simulink model "LW_ctrl"  (R2024b)
settings: Solver=ode4  StartTime=0.0  StopTime=SIM_TIME  FixedStep=0.001  RelTol=1e-3  EnableMultiTasking=on
StartFcn:
  | %timestart = cputime;
StopFcn:
  | %dt = cputime - timestart
undefined symbols (not defined in the file or in its folder): AttCtrl_cycle, ControlMode, DEG2RAD, Earth, FlightMode, LW_ACRO_P_MAX, LW_ACRO_R_MAX, LW_ACRO_Y_MAX, LW_AERO_C0, LW_AERO_C1, LW_AERO_Y0, LW_ANGLE, LW_DMZ0, LW_DMZ_MIN, LW_LAT_CIRCLE, LW_MAN_PITCH_MAX, LW_MAN_ROLL_MAX, LW_MASS, LW_OB_CIRCLE_R, LW_OB_CIRCLE_V, LW_OB_CIRCLE_W, LW_OB_TYPE, LW_REX_YAW, LW_SERVOL_MAX, LW_SERVOR_MAX, LW_THR_HOVER, LW_WZ_MAX, LW_X_ACCEL_MAX, LW_X_ACCEL_MIN, LW_X_FF, LW_X_JERK_MAX, LW_X_P, LW_X_VEL_MAX, LW_Y_ACCEL_MAX, LW_Y_ACCEL_MIN, LW_Y_FF, LW_Y_JERK_MAX, LW_Y_P, LW_Y_VEL_MAX, LW_YAW_KAD, LW_YAW_KAP, LW_Z_ACCEL_LOW, LW_Z_ACCEL_UP, LW_Z_FF, LW_Z_JERK_MAX, LW_Z_P, LW_Z_VEL_MAX_UP, Map_xoffset, Map_yoffset, Map_zoffset, MAX_wdotx, MAX_wdoty, MAX_wdotz, Mixer_cycle, ModelParam_AccelMax, ModelParam_DelayAtt, ModelParam_DelayOmega, ModelParam_DelayPos, ModelParam_envAltitude, ModelParam_envGravityAcc ... (+57)
libraries: pixhawk_slib_uORB_RW x15, simulink x6, slpidlib x6, dspstat3 x5, aerolibnav x4, aerolibtransform2 x3, pixhawk_slib_sensors_actuators x2, etargetslib x2, pixhawk_slib_rfly x1, aerolibatmos2 x1, slrealtimeiplib x1, SignalEditorBlockLib x1
(part 2 of 6)

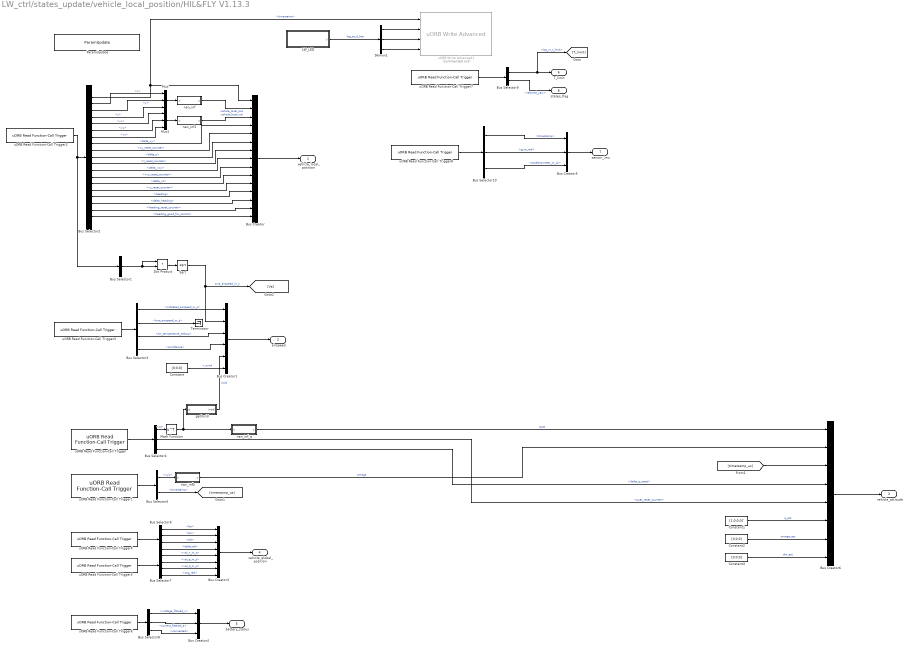
== system LW_ctrl/states_update/vehicle_local_position/HIL&FLY V1.13.3 ==
  Bus Creator : BusCreator  Inputs=15
  Bus Creator1 : BusCreator  Inputs=6
  Bus Creator3 : BusCreator  Inputs=8
  Bus Creator4 : BusCreator  Inputs=3
  Bus Creator5 : BusCreator  Inputs=3
  Bus Creator6 : BusCreator  Inputs=8
  Bus Selector1 : BusSelector  OutputSignals=vx,vy,vz  OutputAsBus=on
  Bus Selector10 : BusSelector  OutputSignals=timestamp,gyro_rad,accelerometer_m_s2
  Bus Selector2 : BusSelector  OutputSignals=timestamp,x,y,z,vx,vy,vz,delta_xy,xy_reset_counter,delta_z,z_reset_counter,delta_vxy,vxy_reset_counter,delta_vz,vz_reset_counter,heading,delta_heading,heading_reset_counter,heading_good_for_control
  Bus Selector3 : BusSelector  OutputSignals=indicated_airspeed_m_s,true_airspeed_m_s,air_temperature_celsius,confidence
  Bus Selector4 : BusSelector  OutputSignals=q,quat_reset_counter,delta_q_reset
  Bus Selector5 : BusSelector  OutputSignals=xyz,timestamp
  Bus Selector6 : BusSelector  OutputSignals=lat,lon,alt,delta_alt
  Bus Selector7 : BusSelector  OutputSignals=vel_n_m_s,vel_e_m_s,vel_d_m_s,cog_rad
  Bus Selector8 : BusSelector  OutputSignals=voltage_filtered_v,current_filtered_a,connected
  Bus Selector9 : BusSelector  OutputSignals=log_m_t_limit,relaxed_yaw
  Constant : Constant  Value=[0;0;0]  OutDataTypeStr=single
  Constant1 : Constant  Value=[1;0;0;0]'  OutDataTypeStr=single
  Constant2 : Constant  Value=[0;0;0]  OutDataTypeStr=single
  Constant3 : Constant  Value=[0;0;0]  OutDataTypeStr=single
  Demux1 : Demux  Outputs=3
  Dot Product : DotProduct  OutDataTypeStr=Inherit: Inherit via internal rule
  LW_LED : MATLAB Function  TreatAsAtomicUnit=on
  Math Function : Math  Operator=transpose
  Mux : Mux  Inputs=3
  Mux1 : Mux  Inputs=3
  ParamUpdate : pixhawk_slib_misc_utils/ParamUpdate  Description=|  Unformatted_StrSet=0  TLC_StrSet=0  NumParams=0  Ts=0
      | ParamUpdate Block
      | 
      | Use this block at your top-level of your model to insert a "parameter update" function in the generated code.
      settings: SourceProductName=Misc Utility Blocks
  Sqrt : Sqrt
  Terminator : Terminator
  getIncid : MATLAB Function  TreatAsAtomicUnit=on
  nan_inf : MATLAB Function  TreatAsAtomicUnit=on
  nan_inf0 : MATLAB Function  TreatAsAtomicUnit=on
  nan_inf1 : MATLAB Function  TreatAsAtomicUnit=on
  nan_inf_q : MATLAB Function  TreatAsAtomicUnit=on
  uORB Read Function-Call Trigger : pixhawk_slib_uORB_RW/uORB Read Function-Call Trigger  uORB_Topic_str='vehicle_attitude'  BusObjVar=Bus: vehicle_attitude_SL  uORB_Interval=0  AsyncOutput=off  Fcn_call_select=Generate Function Call Signal  TaskName='Task1'  Poll_timeout=100  Ts=-1
      settings: SourceProductName=uORB Read / Write Blocks
  uORB Read Function-Call Trigger1 : pixhawk_slib_uORB_RW/uORB Read Function-Call Trigger  uORB_Topic_str='vehicle_angular_velocity'  BusObjVar=Bus: vehicle_angular_velocity_SL  uORB_Interval=0  AsyncOutput=off  Fcn_call_select=Generate Function Call Signal  TaskName='Task1'  Poll_timeout=100  Ts=-1
      settings: SourceProductName=uORB Read / Write Blocks
  uORB Read Function-Call Trigger2 : pixhawk_slib_uORB_RW/uORB Read Function-Call Trigger  Priority=2  uORB_Topic_str='vehicle_local_position'  BusObjVar=Bus: vehicle_local_position_SL  uORB_Interval=0  AsyncOutput=off  Fcn_call_select=Generate Function Call Signal  TaskName='Task2'  Poll_timeout=20  Ts=-1
      settings: SourceProductName=uORB Read / Write Blocks
  uORB Read Function-Call Trigger3 : pixhawk_slib_uORB_RW/uORB Read Function-Call Trigger  Priority=2  uORB_Topic_str='airspeed'  BusObjVar=Bus: airspeed_SL  uORB_Interval=0  AsyncOutput=off  Fcn_call_select=Generate Function Call Signal  TaskName='Task2'  Poll_timeout=20  Ts=-1
      settings: SourceProductName=uORB Read / Write Blocks
  uORB Read Function-Call Trigger4 : pixhawk_slib_uORB_RW/uORB Read Function-Call Trigger  Priority=2  uORB_Topic_str='vehicle_global_position'  BusObjVar=Bus: vehicle_global_position_SL  uORB_Interval=0  AsyncOutput=off  Fcn_call_select=Generate Function Call Signal  TaskName='Task2'  Poll_timeout=20  Ts=-1
      settings: SourceProductName=uORB Read / Write Blocks
  uORB Read Function-Call Trigger5 : pixhawk_slib_uORB_RW/uORB Read Function-Call Trigger  Priority=2  uORB_Topic_str='vehicle_gps_position'  BusObjVar=Bus: vehicle_gps_position_SL  uORB_Interval=0  AsyncOutput=off  Fcn_call_select=Generate Function Call Signal  TaskName='Task2'  Poll_timeout=20  Ts=-1
      settings: SourceProductName=uORB Read / Write Blocks
  uORB Read Function-Call Trigger6 : pixhawk_slib_uORB_RW/uORB Read Function-Call Trigger  Priority=2  uORB_Topic_str='battery_status'  BusObjVar=Bus: battery_status_SL  uORB_Interval=0  AsyncOutput=off  Fcn_call_select=Generate Function Call Signal  TaskName='Task2'  Poll_timeout=20  Ts=-1
      settings: SourceProductName=uORB Read / Write Blocks
  uORB Read Function-Call Trigger7 : pixhawk_slib_uORB_RW/uORB Read Function-Call Trigger  Priority=2  uORB_Topic_str='costom_lw_mixer'  BusObjVar=Bus: costom_lw_mixer_SL  uORB_Interval=0  AsyncOutput=off  Fcn_call_select=Generate Function Call Signal  TaskName='Task2'  Poll_timeout=20  Ts=-1
      settings: SourceProductName=uORB Read / Write Blocks
  uORB Read Function-Call Trigger8 : pixhawk_slib_uORB_RW/uORB Read Function-Call Trigger  Priority=2  uORB_Topic_str='sensor_combined'  BusObjVar=Bus: sensor_combined_SL  uORB_Interval=0  AsyncOutput=off  Fcn_call_select=Generate Function Call Signal  TaskName='Task2'  Poll_timeout=20  Ts=-1
      settings: SourceProductName=uORB Read / Write Blocks
  uORB Write Advanced1 : pixhawk_slib_uORB_RW/uORB Write Advanced  Commented=on  Ts=0  uORB_AdvtQueue=on  uORB_FieldEnabledArr="0  0  0  1  0  0  0  0  0  0  0"  uORB_Topic_str=0  uORB_Struct_DT="[1  1  1  1  1]"  BlockInputCount=5  uORB_StructParams="[\"voltage_v\",\"voltage_filtered_v\",\"current_a\",\"current_filtered_a\",\"remaining\"]"  uORB_PortSizes="[1  1  1  1]"  MsgSizeOf=0  MW_update=true
      settings: SourceProductName=uORB Read / Write Blocks
  vehicle_local_position : Outport  VectorParamsAs1DForOutWhenUnconnected=off
  airspeed : Outport  Port=2  VectorParamsAs1DForOutWhenUnconnected=off
  vehicle_attitude : Outport  Port=3  VectorParamsAs1DForOutWhenUnconnected=off
  vehicle_global_position : Outport  Port=4  OutDataTypeStr=Bus: vehicle_global_position_bus  VectorParamsAs1DForOutWhenUnconnected=off
  battery_status : Outport  Port=5  OutDataTypeStr=Bus: battery_status_bus  VectorParamsAs1DForOutWhenUnconnected=off
  T_limit : Outport  Port=6  VectorParamsAs1DForOutWhenUnconnected=off
  sensor_imu : Outport  Port=7  VectorParamsAs1DForOutWhenUnconnected=off
  states_flag : Outport  Port=8  VectorParamsAs1DForOutWhenUnconnected=off
  wires:
  Bus Selector1/1 -> Dot Product/1, Dot Product/2
  Bus Selector2/6 -> Mux1/2  "<vy>"
  Bus Selector2/3 -> Mux/2  "<y>"
  uORB Read Function-Call Trigger2/1 -> Bus Selector1/1, Bus Selector2/1
  uORB Read Function-Call Trigger3/1 -> Bus Selector3/1
  Sqrt/1 -> Bus Creator1/2, [Va]  "true_airspeed_m_s"
  Bus Selector2/2 -> Mux/1  "<x>"
  Bus Selector8/1 -> Bus Creator4/1  "<voltage_filtered_v>"
  Bus Selector10/1 -> Bus Creator5/1  "<timestamp>"
  Bus Selector7/1 -> Bus Creator3/5  "<vel_n_m_s>"
  Dot Product/1 -> Sqrt/1
  Mux/1 -> nan_inf/1(u)
  Bus Creator5/1 -> sensor_imu/1
  Bus Selector10/3 -> Bus Creator5/3  "<accelerometer_m_s2>"
  uORB Read Function-Call Trigger6/1 -> Bus Selector8/1
  Bus Selector2/4 -> Mux/3  "<z>"
  Bus Creator/1 -> vehicle_local_position/1
  Bus Selector6/3 -> Bus Creator3/3  "<alt>"
  Bus Selector10/2 -> Bus Creator5/2  "<gyro_rad>"
  Bus Selector9/1 -> [T_limit], T_limit/1  "<log_m_t_limit>"
  Constant/1 -> Bus Creator1/6  "v_wind"
  Mux1/1 -> nan_inf1/1(u)
  nan_inf/1(y) -> Bus Creator/2  "vehicle_local_pos"
  Bus Selector7/3 -> Bus Creator3/7  "<vel_d_m_s>"
  uORB Read Function-Call Trigger5/1 -> Bus Selector7/1
  Bus Selector2/5 -> Mux1/1  "<vx>"
  uORB Read Function-Call Trigger4/1 -> Bus Selector6/1
  uORB Read Function-Call Trigger8/1 -> Bus Selector10/1
  Bus Selector6/1 -> Bus Creator3/1  "<lat>"
  Bus Selector2/7 -> Mux1/3  "<vz>"
  Bus Selector8/3 -> Bus Creator4/3  "<connected>"
  getIncid/1(incid) -> Bus Creator1/5  "incid"
  Bus Selector4/1 -> Math Function/1  "<q>"
  Bus Selector6/4 -> Bus Creator3/4  "<delta_alt>"
  nan_inf_q/1(y) -> Bus Creator6/1  "quat"
  Bus Selector7/4 -> Bus Creator3/8  "<cog_rad>"
  uORB Read Function-Call Trigger1/1 -> Bus Selector5/1
  Bus Creator1/1 -> airspeed/1
  Bus Selector3/3 -> Bus Creator1/3  "<air_temperature_celsius>"
  Bus Selector5/1 -> nan_inf0/1(u)  "<xyz>"
  Math Function/1 -> getIncid/1(q), nan_inf_q/1(u)
  Bus Selector6/2 -> Bus Creator3/2  "<lon>"
  Bus Creator3/1 -> vehicle_global_position/1
  Bus Selector7/2 -> Bus Creator3/6  "<vel_e_m_s>"
  Bus Selector9/2 -> states_flag/1  "<relaxed_yaw>"
  Bus Selector3/1 -> Bus Creator1/1  "<indicated_airspeed_m_s>"
  Bus Creator4/1 -> battery_status/1
  Bus Selector8/2 -> Bus Creator4/2  "<current_filtered_a>"
  uORB Read Function-Call Trigger/1 -> Bus Selector4/1
  nan_inf1/1(y) -> Bus Creator/3  "vehicle_local_vel"
  uORB Read Function-Call Trigger7/1 -> Bus Selector9/1
  Bus Selector5/2 -> [timestamp_us]  "<timestamp>"
  Bus Selector3/2 -> Terminator/1  "<true_airspeed_m_s>"
  Bus Selector3/4 -> Bus Creator1/4  "<confidence>"
  Bus Selector2/1 -> Bus Creator/1, uORB Write Advanced1/1  "<timestamp>"
  Demux1/2 -> uORB Write Advanced1/3
  Demux1/3 -> uORB Write Advanced1/4
  Demux1/1 -> uORB Write Advanced1/2
  LW_LED/1(y) -> Demux1/1  "log_ac_d_hat"
  Bus Selector2/8 -> Bus Creator/4  "<delta_xy>"
  Bus Selector2/9 -> Bus Creator/5  "<xy_reset_counter>"
  Bus Selector2/10 -> Bus Creator/6  "<delta_z>"
  Bus Selector2/11 -> Bus Creator/7  "<z_reset_counter>"
  Bus Selector2/12 -> Bus Creator/8  "<delta_vxy>"
  Bus Selector2/13 -> Bus Creator/9  "<vxy_reset_counter>"
  Bus Selector2/14 -> Bus Creator/10  "<delta_vz>"
  Bus Selector2/15 -> Bus Creator/11  "<vz_reset_counter>"
  Bus Selector2/16 -> Bus Creator/12  "<heading>"
  Bus Selector2/17 -> Bus Creator/13  "<delta_heading>"
  Bus Selector2/18 -> Bus Creator/14  "<heading_reset_counter>"
  Bus Selector2/19 -> Bus Creator/15  "<heading_good_for_control>"
  [timestamp_us] -> Bus Creator6/3
  Bus Creator6/1 -> vehicle_attitude/1
  Bus Selector4/2 -> Bus Creator6/5  "<quat_reset_counter>"
  nan_inf0/1(y) -> Bus Creator6/2  "omega"
  Bus Selector4/3 -> Bus Creator6/4  "<delta_q_reset>"
  Constant1/1 -> Bus Creator6/6  "q_est"
  Constant2/1 -> Bus Creator6/7  "omega_est"
  Constant3/1 -> Bus Creator6/8  "dm_est"

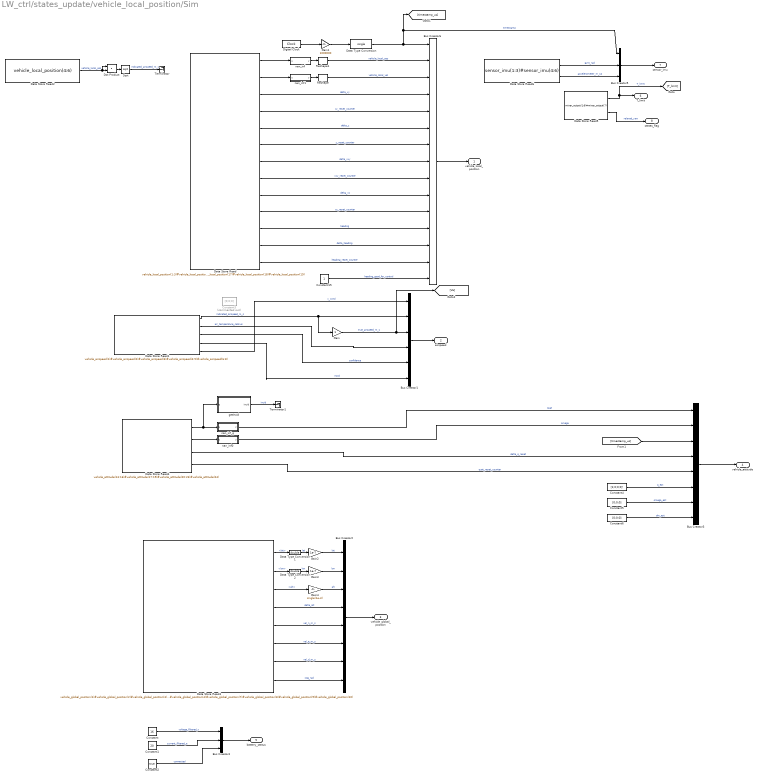
== system LW_ctrl/states_update/vehicle_local_position/Sim ==
  Bus Creator1 : BusCreator  Inputs=6
  Bus Creator2 : BusCreator  Inputs=8
  Bus Creator3 : BusCreator  Inputs=8
  Bus Creator4 : BusCreator  Inputs=3
  Bus Creator5 : BusCreator  Inputs=3
  Bus Creator6 : BusCreator  Inputs=15
  Constant : Constant  Value=16  OutDataTypeStr=single
  Constant1 : Constant  Value=20  OutDataTypeStr=single
  Constant15 : Constant  OutDataTypeStr=boolean
  Constant2 : Constant  Value=true  OutDataTypeStr=boolean
  Constant3 : Constant  Commented=on  Value=[0;0;0]  OutDataTypeStr=single
  Constant4 : Constant  Value=[1;0;0;0]'  OutDataTypeStr=single
  Constant5 : Constant  Value=[0;0;0]  OutDataTypeStr=single
  Constant6 : Constant  Value=[0;0;0]  OutDataTypeStr=single
  Data Store Read : DataStoreRead  DataStoreName=vehicle_local_position  DataStoreElements=vehicle_local_position(1:3)#vehicle_local_position(4:6)#vehicle_local_position(7:8)#vehicle_local_position(9)#vehicle_local_position(10)#vehicle_local_position(11)#vehicle_local_position(12:13)#vehicle_local_position(14)#vehicle_local_position(15)#vehicle_local_position(16)#vehicle_local_position(17)#vehicle_local_position(18)#vehicle_local_position(19)  IndexOptions=Index vector (dialog)  Indices=1  OutputSizes=1
  Data Store Read1 : DataStoreRead  DataStoreName=vehicle_airspeed  DataStoreElements=vehicle_airspeed(1)#vehicle_airspeed(2)#vehicle_airspeed(3)#vehicle_airspeed(4:5)#vehicle_airspeed(6:8)  IndexOptions=Index vector (dialog)  Indices=1  OutputSizes=1
  Data Store Read2 : DataStoreRead  DataStoreName=vehicle_local_position  DataStoreElements=vehicle_local_position(4:6)  IndexOptions=Index vector (dialog)  Indices=1  OutputSizes=1
  Data Store Read3 : DataStoreRead  DataStoreName=vehicle_global_position  DataStoreElements=vehicle_global_position(1)#vehicle_global_position(2)#vehicle_global_position(3)#vehicle_global_position(4)#vehicle_global_position(7)#vehicle_global_position(8)#vehicle_global_position(9)#vehicle_global_position(10)  IndexOptions=Index vector (dialog)  Indices=1  OutputSizes=1
  Data Store Read4 : DataStoreRead  DataStoreName=vehicle_attitude  DataStoreElements=vehicle_attitude(13:16)#vehicle_attitude(17:19)#vehicle_attitude(20:23)#vehicle_attitude(24)  IndexOptions=Index vector (dialog)  Indices=1  OutputSizes=1
  Data Store Read5 : DataStoreRead  Description=|  DataStoreName=mixer_output  DataStoreElements=mixer_output(1:6)#mixer_output(7)  IndexOptions=Index vector (dialog)  Indices=1  OutputSizes=1
      | 1-4:motor command
      | 5-6:aileron command
  Data Store Read6 : DataStoreRead  DataStoreName=sensor_imu  DataStoreElements=sensor_imu(1:3)#sensor_imu(4:6)  IndexOptions=Index vector (dialog)  Indices=1  OutputSizes=1
  Data Type Conversion : DataTypeConversion  OutDataTypeStr=single  SaturateOnIntegerOverflow=off  RndMeth=Floor
  Data Type Conversion1 : DataTypeConversion  OutDataTypeStr=double  SaturateOnIntegerOverflow=off  RndMeth=Floor
  Data Type Conversion2 : DataTypeConversion  OutDataTypeStr=double  SaturateOnIntegerOverflow=off  RndMeth=Floor
  Digital Clock : DigitalClock  SampleTime=-1
  Dot Product : DotProduct  OutDataTypeStr=Inherit: Inherit via internal rule
  Gain : Gain
  Gain1 : Gain  Gain=1000000
  Gain2 : Gain  Gain=1e-7  OutDataTypeStr=double
  Gain3 : Gain  Gain=1e-7  OutDataTypeStr=double
  Gain4 : Gain  Gain=single(1e-3)  OutDataTypeStr=single
  Reshape : Reshape  OutputDimensionality=Column vector (2-D)
  Reshape1 : Reshape  OutputDimensionality=Column vector (2-D)
  Sqrt : Sqrt
  Terminator : Terminator
  Terminator1 : Terminator
  getIncid : MATLAB Function  TreatAsAtomicUnit=on
  nan_inf : MATLAB Function  TreatAsAtomicUnit=on
  nan_inf0 : MATLAB Function  TreatAsAtomicUnit=on
  nan_inf1 : MATLAB Function  TreatAsAtomicUnit=on
  nan_inf_q : MATLAB Function  TreatAsAtomicUnit=on
  vehicle_local_position : Outport  VectorParamsAs1DForOutWhenUnconnected=off
  airspeed : Outport  Port=2  VectorParamsAs1DForOutWhenUnconnected=off
  vehicle_global_position : Outport  Port=3  OutDataTypeStr=Bus: vehicle_global_position_bus  VectorParamsAs1DForOutWhenUnconnected=off
  vehicle_attitude : Outport  Port=4  VectorParamsAs1DForOutWhenUnconnected=off
  battery_status : Outport  Port=5  OutDataTypeStr=Bus: battery_status_bus  VectorParamsAs1DForOutWhenUnconnected=off
  T_limit : Outport  Port=6  VectorParamsAs1DForOutWhenUnconnected=off
  sensor_imu : Outport  Port=7  VectorParamsAs1DForOutWhenUnconnected=off
  states_flag : Outport  Port=8  VectorParamsAs1DForOutWhenUnconnected=off
  wires:
  Data Store Read/1 -> nan_inf/1(u)
  Data Store Read/2 -> nan_inf1/1(u)
  nan_inf/1(y) -> Reshape1/1
  nan_inf1/1(y) -> Reshape/1
  Digital Clock/1 -> Gain1/1
  Reshape/1 -> Bus Creator6/3  "vehicle_local_vel"
  Reshape1/1 -> Bus Creator6/2  "vehicle_local_pos"
  Data Store Read1/3 -> Bus Creator1/5  "confidence"
  Data Store Read1/2 -> Bus Creator1/4  "air_temperature_celsius"
  Data Store Read2/1 -> Dot Product/2, Dot Product/1  "vehicle_local_pos"
  Dot Product/1 -> Sqrt/1
  Sqrt/1 -> Terminator/1  "indicated_airspeed_m_s"
  Gain/1 -> [Va], Bus Creator1/3  "true_airspeed_m_s"
  Bus Creator1/1 -> airspeed/1
  Data Store Read1/1 -> Bus Creator1/2, Gain/1  "indicated_airspeed_m_s"
  Data Store Read3/5 -> Bus Creator2/5  "vel_n_m_s"
  Gain3/1 -> Bus Creator2/2  "lon"
  Gain2/1 -> Bus Creator2/1  "lat"
  Data Store Read3/8 -> Bus Creator2/8  "cog_rad"
  Data Store Read3/3 -> Gain4/1  "<alt>"
  Data Store Read3/4 -> Bus Creator2/4  "delta_alt"
  Data Store Read3/6 -> Bus Creator2/6  "vel_e_m_s"
  Data Store Read3/1 -> Data Type Conversion1/1  "<lat>"
  Data Store Read3/7 -> Bus Creator2/7  "vel_d_m_s"
  Bus Creator2/1 -> vehicle_global_position/1
  Gain4/1 -> Bus Creator2/3  "alt"
  Data Store Read3/2 -> Data Type Conversion2/1  "<lon>"
  Data Store Read4/1 -> nan_inf_q/1(u), getIncid/1(q)
  Bus Creator3/1 -> vehicle_attitude/1
  Data Store Read4/2 -> nan_inf0/1(u)
  Data Store Read1/4 -> Bus Creator1/6  "incid"
  Gain1/1 -> Data Type Conversion/1
  Data Type Conversion1/1 -> Gain2/1  "lat"
  Data Type Conversion2/1 -> Gain3/1  "lon"
  getIncid/1(incid) -> Terminator1/1  "incid"
  Constant1/1 -> Bus Creator4/2  "current_filtered_a"
  Constant/1 -> Bus Creator4/1  "voltage_filtered_v"
  Bus Creator4/1 -> battery_status/1
  Constant2/1 -> Bus Creator4/3  "connected"
  Data Store Read5/1 -> [T_limit], T_limit/1  "T_limit"
  Data Store Read1/5 -> Bus Creator1/1  "v_wind"
  Bus Creator5/1 -> sensor_imu/1
  Data Store Read6/2 -> Bus Creator5/3  "accelerometer_m_s2"
  Data Store Read6/1 -> Bus Creator5/2  "gyro_rad"
  Data Type Conversion/1 -> [timestamp_us], Bus Creator5/1, Bus Creator6/1  "timestamp"
  Data Store Read5/2 -> states_flag/1  "relaxed_yaw"
  Data Store Read/4 -> Bus Creator6/5  "xy_reset_counter"
  Data Store Read/3 -> Bus Creator6/4  "delta_xy"
  Data Store Read/9 -> Bus Creator6/10  "delta_vz"
  Data Store Read/5 -> Bus Creator6/6  "delta_z"
  Data Store Read/12 -> Bus Creator6/13  "delta_heading"
  Data Store Read/13 -> Bus Creator6/14  "heading_reset_counter"
  Data Store Read/11 -> Bus Creator6/12  "heading"
  Data Store Read/6 -> Bus Creator6/7  "z_reset_counter"
  Constant15/1 -> Bus Creator6/15  "heading_good_for_control"
  Data Store Read/10 -> Bus Creator6/11  "vz_reset_counter"
  Data Store Read/8 -> Bus Creator6/9  "vxy_reset_counter"
  Data Store Read/7 -> Bus Creator6/8  "delta_vxy"
  Bus Creator6/1 -> vehicle_local_position/1
  Data Store Read4/3 -> Bus Creator3/4  "delta_q_reset"
  nan_inf0/1(y) -> Bus Creator3/2  "omega"
  Data Store Read4/4 -> Bus Creator3/5  "quat_reset_counter"
  nan_inf_q/1(y) -> Bus Creator3/1  "quat"
  [timestamp_us] -> Bus Creator3/3
  Constant6/1 -> Bus Creator3/8  "dm_est"
  Constant4/1 -> Bus Creator3/6  "q_est"
  Constant5/1 -> Bus Creator3/7  "omega_est"

== system LW_ctrl/Controller/PID_Controller/PID_Controller/altitude control ==
  p : Inport
  q : Inport  Port=2
  attitude_d : Inport  Port=3
  r : Inport  Port=4
  f_d : Inport  Port=5
  quat : Inport  Port=6
  vehicle_mode : Inport  Port=7
  Bus Selector3 : BusSelector  OutputSignals=flight_mode,arm,ctrl_mode
  Cast To Single : DataTypeConversion  OutDataTypeStr=single  SaturateOnIntegerOverflow=off  RndMeth=Floor
  MATLAB Function : MATLAB Function
  MATLAB Function1 : MATLAB Function
  Mux12 : Mux
  Output_Limits1 : Saturate  UpperLimit=15  LowerLimit=0
  Selector1 : Selector  InputPortWidth=3  IndexOptions=Index vector (dialog)  Indices=[1]  OutputSizes=1
  Selector2 : Selector  InputPortWidth=3  IndexOptions=Index vector (dialog)  Indices=3  OutputSizes=1
  Selector3 : Selector  InputPortWidth=3  IndexOptions=Index vector (dialog)  Indices=2  OutputSizes=1
  Sum : Sum  Inputs=|+-
  Sum2 : Sum  Inputs=|+-
  Sum3 : Sum  Inputs=|+-
  attrates_ref_selector : MATLAB Function  TreatAsAtomicUnit=on
  wx_control : slpidlib/PID Controller  Controller=PID  Form=Parallel  TimeDomain=Discrete-time  UseExternalTs=off  SampleTime=-1  IntegratorMethod=Forward Euler  FilterMethod=Forward Euler  ControllerParametersSource=internal  P=20  I=0  UseKiTs=off  D=0  UseExternalDerivativeSource=off  N=100  UseFilter=on  TunerSelectOption=Transfer Function Based (PID Tuner App)  InitialConditionSource=internal  InitialConditionForIntegrator=0  InitialConditionForFilter=0  DifferentiatorICPrevScaledInput=0  ExternalReset=level  TrackingMode=off  Kt=1  LimitOutput=on  SatLimitsSource=internal  UpperSaturationLimit=MAX_wdotx  LowerSaturationLimit=-MAX_wdotx  LinearizeAsGain=off  AntiWindupMode=clamping  Kb=1  LimitIntegrator=off  UpperIntegratorSaturationLimit=inf  LowerIntegratorSaturationLimit=-inf  POutMin=[]  POutMax=[]  IOutMin=[]  IOutMax=[]  DOutMin=[]  DOutMax=[]  NOutMin=[]  NOutMax=[]  SumOutMin=[]  SumOutMax=[]  SaturationOutMin=[]  SaturationOutMax=[]  PParamMin=[]  PParamMax=[]  IParamMin=[]  IParamMax=[]  DParamMin=[]  DParamMax=[]  NParamMin=[]  NParamMax=[]  KbParamMin=[]  KbParamMax=[]  KtParamMin=[]  KtParamMax=[]  KbOutMin=[]  KbOutMax=[]  KtOutMin=[]  KtOutMax=[]  IntegratorOutMin=Saturation_I_Wx_Low  IntegratorOutMax=Saturation_I_Wx_Up  FilterOutMin=[]  FilterOutMax=[]  SumI1OutMin=[]  SumI1OutMax=[]  SumI2OutMin=[]  SumI2OutMax=[]  SumI3OutMin=[]  SumI3OutMax=[]  SumI4OutMin=[]  SumI4OutMax=[]  SumDOutMin=[]  SumDOutMax=[]  DifferentiatorOutMin=[]  DifferentiatorOutMax=[]  FilterDiffOutCoefMin=[]  FilterDiffOutCoefMax=[]  ReciprocalOutMin=[]  ReciprocalOutMax=[]  SumDenOutMin=[]  SumDenOutMax=[]  SumNumOutMin=[]  SumNumOutMax=[]  DivideOutMin=[]  DivideOutMax=[]  UdiffTsProdOutMin=[]  UdiffTsProdOutMax=[]  NTsProdOutMin=[]  NTsProdOutMax=[]  UintegralTsProdOutMin=[]  UintegralTsProdOutMax=[]  UngainTsProdOutMin=[]  UngainTsProdOutMax=[]  ClampingZeroOutDataTypeStr=Inherit: Inherit via back propagation  ClampingZeroOutMin=[]  ClampingZeroOutMax=[]  FilterDenConstantOutDataTypeStr=Inherit: Inherit via back propagation  FilterDenConstantOutMin=[]  FilterDenConstantOutMax=[]  PCopyOutDataTypeStr=Inherit: Inherit via back propagation  PCopyOutMin=[]  PCopyOutMax=[]  NCopyOutDataTypeStr=Inherit: Inherit via back propagation  NCopyOutMin=[]  NCopyOutMax=[]  IntegratorContinuousStateAttributes=''  IntegratorStateMustResolveToSignalObject=off  IntegratorRTWStateStorageClass=Auto  FilterContinuousStateAttributes=''  FilterStateMustResolveToSignalObject=off  FilterRTWStateStorageClass=Auto  ParallelPVariant=InternalParameters  IdealPVariant=Disabled  IVariant=InternalParameters  DVariant=InternalParameters  IntegratorVariant=Discrete  SatVariant=Enabled  AWVariant=DiscClampingParallel  PCopyVariant=Disabled  TRVariant=Disabled  FdbkBlocksVariant=Forward  IdealPFdbkVariant=Disabled  SatFdbkVariant=Disabled  DerivativeFilterVariant=ForwardEulerFilter  NVariant=InternalParameters  NCopyVariant=Disabled  FilterICVariant=InternalICsFilter  IntegratorICVariant=InternalICs  ExternalResetVariant=ExternalReset  TRSumVariant=Passthrough  SumFdbkVariant=Disabled  SumVariant=Sum_PID  TsampFilterVariant=InternalTs  TsampNgainVariant=Passthrough  TsampIntegralVariant=Disabled_SignalSpec  ExternalSaturationOutDataTypeStr=Inherit: Same as second input  DerivativeSourceVariant=ErrorSignal  PreIntVariant=InternalPreInt
  wy_control : slpidlib/PID Controller  Controller=PID  Form=Parallel  TimeDomain=Discrete-time  UseExternalTs=off  SampleTime=-1  IntegratorMethod=Forward Euler  FilterMethod=Forward Euler  ControllerParametersSource=internal  P=20  I=0  UseKiTs=off  D=0  UseExternalDerivativeSource=off  N=100  UseFilter=on  TunerSelectOption=Transfer Function Based (PID Tuner App)  InitialConditionSource=internal  InitialConditionForIntegrator=0  InitialConditionForFilter=0  DifferentiatorICPrevScaledInput=0  ExternalReset=level  TrackingMode=off  Kt=1  LimitOutput=on  SatLimitsSource=internal  UpperSaturationLimit=MAX_wdoty  LowerSaturationLimit=-MAX_wdoty  LinearizeAsGain=off  AntiWindupMode=clamping  Kb=1  LimitIntegrator=off  UpperIntegratorSaturationLimit=inf  LowerIntegratorSaturationLimit=-inf  POutMin=[]  POutMax=[]  IOutMin=[]  IOutMax=[]  DOutMin=[]  DOutMax=[]  NOutMin=[]  NOutMax=[]  SumOutMin=[]  SumOutMax=[]  SaturationOutMin=[]  SaturationOutMax=[]  PParamMin=[]  PParamMax=[]  IParamMin=[]  IParamMax=[]  DParamMin=[]  DParamMax=[]  NParamMin=[]  NParamMax=[]  KbParamMin=[]  KbParamMax=[]  KtParamMin=[]  KtParamMax=[]  KbOutMin=[]  KbOutMax=[]  KtOutMin=[]  KtOutMax=[]  IntegratorOutMin=Saturation_I_Wy_Low  IntegratorOutMax=Saturation_I_Wy_Up  FilterOutMin=[]  FilterOutMax=[]  SumI1OutMin=[]  SumI1OutMax=[]  SumI2OutMin=[]  SumI2OutMax=[]  SumI3OutMin=[]  SumI3OutMax=[]  SumI4OutMin=[]  SumI4OutMax=[]  SumDOutMin=[]  SumDOutMax=[]  DifferentiatorOutMin=[]  DifferentiatorOutMax=[]  FilterDiffOutCoefMin=[]  FilterDiffOutCoefMax=[]  ReciprocalOutMin=[]  ReciprocalOutMax=[]  SumDenOutMin=[]  SumDenOutMax=[]  SumNumOutMin=[]  SumNumOutMax=[]  DivideOutMin=[]  DivideOutMax=[]  UdiffTsProdOutMin=[]  UdiffTsProdOutMax=[]  NTsProdOutMin=[]  NTsProdOutMax=[]  UintegralTsProdOutMin=[]  UintegralTsProdOutMax=[]  UngainTsProdOutMin=[]  UngainTsProdOutMax=[]  ClampingZeroOutDataTypeStr=Inherit: Inherit via back propagation  ClampingZeroOutMin=[]  ClampingZeroOutMax=[]  FilterDenConstantOutDataTypeStr=Inherit: Inherit via back propagation  FilterDenConstantOutMin=[]  FilterDenConstantOutMax=[]  PCopyOutDataTypeStr=Inherit: Inherit via back propagation  PCopyOutMin=[]  PCopyOutMax=[]  NCopyOutDataTypeStr=Inherit: Inherit via back propagation  NCopyOutMin=[]  NCopyOutMax=[]  IntegratorContinuousStateAttributes=''  IntegratorStateMustResolveToSignalObject=off  IntegratorRTWStateStorageClass=Auto  FilterContinuousStateAttributes=''  FilterStateMustResolveToSignalObject=off  FilterRTWStateStorageClass=Auto  ParallelPVariant=InternalParameters  IdealPVariant=Disabled  IVariant=InternalParameters  DVariant=InternalParameters  IntegratorVariant=Discrete  SatVariant=Enabled  AWVariant=DiscClampingParallel  PCopyVariant=Disabled  TRVariant=Disabled  FdbkBlocksVariant=Forward  IdealPFdbkVariant=Disabled  SatFdbkVariant=Disabled  DerivativeFilterVariant=ForwardEulerFilter  NVariant=InternalParameters  NCopyVariant=Disabled  FilterICVariant=InternalICsFilter  IntegratorICVariant=InternalICs  ExternalResetVariant=ExternalReset  TRSumVariant=Passthrough  SumFdbkVariant=Disabled  SumVariant=Sum_PID  TsampFilterVariant=InternalTs  TsampNgainVariant=Passthrough  TsampIntegralVariant=Disabled_SignalSpec  ExternalSaturationOutDataTypeStr=Inherit: Same as second input  DerivativeSourceVariant=ErrorSignal  PreIntVariant=InternalPreInt
  wz_control : slpidlib/PID Controller  Controller=PID  Form=Parallel  TimeDomain=Discrete-time  UseExternalTs=off  SampleTime=-1  IntegratorMethod=Forward Euler  FilterMethod=Forward Euler  ControllerParametersSource=internal  P=20  I=0  UseKiTs=off  D=0  UseExternalDerivativeSource=off  N=100  UseFilter=on  TunerSelectOption=Transfer Function Based (PID Tuner App)  InitialConditionSource=internal  InitialConditionForIntegrator=0  InitialConditionForFilter=0  DifferentiatorICPrevScaledInput=0  ExternalReset=level  TrackingMode=off  Kt=1  LimitOutput=on  SatLimitsSource=internal  UpperSaturationLimit=MAX_wdotz  LowerSaturationLimit=-MAX_wdotz  LinearizeAsGain=off  AntiWindupMode=clamping  Kb=1  LimitIntegrator=off  UpperIntegratorSaturationLimit=inf  LowerIntegratorSaturationLimit=-inf  POutMin=[]  POutMax=[]  IOutMin=[]  IOutMax=[]  DOutMin=[]  DOutMax=[]  NOutMin=[]  NOutMax=[]  SumOutMin=[]  SumOutMax=[]  SaturationOutMin=[]  SaturationOutMax=[]  PParamMin=[]  PParamMax=[]  IParamMin=[]  IParamMax=[]  DParamMin=[]  DParamMax=[]  NParamMin=[]  NParamMax=[]  KbParamMin=[]  KbParamMax=[]  KtParamMin=[]  KtParamMax=[]  KbOutMin=[]  KbOutMax=[]  KtOutMin=[]  KtOutMax=[]  IntegratorOutMin=Saturation_I_Wz_Low  IntegratorOutMax=Saturation_I_Wz_Up  FilterOutMin=[]  FilterOutMax=[]  SumI1OutMin=[]  SumI1OutMax=[]  SumI2OutMin=[]  SumI2OutMax=[]  SumI3OutMin=[]  SumI3OutMax=[]  SumI4OutMin=[]  SumI4OutMax=[]  SumDOutMin=[]  SumDOutMax=[]  DifferentiatorOutMin=[]  DifferentiatorOutMax=[]  FilterDiffOutCoefMin=[]  FilterDiffOutCoefMax=[]  ReciprocalOutMin=[]  ReciprocalOutMax=[]  SumDenOutMin=[]  SumDenOutMax=[]  SumNumOutMin=[]  SumNumOutMax=[]  DivideOutMin=[]  DivideOutMax=[]  UdiffTsProdOutMin=[]  UdiffTsProdOutMax=[]  NTsProdOutMin=[]  NTsProdOutMax=[]  UintegralTsProdOutMin=[]  UintegralTsProdOutMax=[]  UngainTsProdOutMin=[]  UngainTsProdOutMax=[]  ClampingZeroOutDataTypeStr=Inherit: Inherit via back propagation  ClampingZeroOutMin=[]  ClampingZeroOutMax=[]  FilterDenConstantOutDataTypeStr=Inherit: Inherit via back propagation  FilterDenConstantOutMin=[]  FilterDenConstantOutMax=[]  PCopyOutDataTypeStr=Inherit: Inherit via back propagation  PCopyOutMin=[]  PCopyOutMax=[]  NCopyOutDataTypeStr=Inherit: Inherit via back propagation  NCopyOutMin=[]  NCopyOutMax=[]  IntegratorContinuousStateAttributes=''  IntegratorStateMustResolveToSignalObject=off  IntegratorRTWStateStorageClass=Auto  FilterContinuousStateAttributes=''  FilterStateMustResolveToSignalObject=off  FilterRTWStateStorageClass=Auto  ParallelPVariant=InternalParameters  IdealPVariant=Disabled  IVariant=InternalParameters  DVariant=InternalParameters  IntegratorVariant=Discrete  SatVariant=Enabled  AWVariant=DiscClampingParallel  PCopyVariant=Disabled  TRVariant=Disabled  FdbkBlocksVariant=Forward  IdealPFdbkVariant=Disabled  SatFdbkVariant=Disabled  DerivativeFilterVariant=ForwardEulerFilter  NVariant=InternalParameters  NCopyVariant=Disabled  FilterICVariant=InternalICsFilter  IntegratorICVariant=InternalICs  ExternalResetVariant=ExternalReset  TRSumVariant=Passthrough  SumFdbkVariant=Disabled  SumVariant=Sum_PID  TsampFilterVariant=InternalTs  TsampNgainVariant=Passthrough  TsampIntegralVariant=Disabled_SignalSpec  ExternalSaturationOutDataTypeStr=Inherit: Same as second input  DerivativeSourceVariant=ErrorSignal  PreIntVariant=InternalPreInt
  T : Outport
  wires:
  Mux12/1 -> Output_Limits1/1
  Output_Limits1/1 -> T/1
  r/1 -> Sum2/2
  p/1 -> Sum3/2
  Cast To Single/1 -> MATLAB Function/1(f_d)
  q/1 -> Sum/2
  f_d/1 -> Cast To Single/1
  quat/1 -> MATLAB Function1/1(quat)
  MATLAB Function/1(T1) -> Mux12/1
  MATLAB Function/2(T2) -> Mux12/2
  MATLAB Function/3(T3) -> Mux12/3
  MATLAB Function/4(T4) -> Mux12/4
  MATLAB Function1/1(psi_err) -> Sum2/1
  MATLAB Function1/2(phi_err) -> Sum3/1
  MATLAB Function1/3(theta_err) -> Sum/1
  Selector1/1 -> wx_control/2  "reset_x"
  Selector3/1 -> wy_control/2  "reset_y"
  Selector2/1 -> wz_control/2  "reset_z"
  Sum3/1 -> wx_control/1
  wx_control/1 -> MATLAB Function/2(Mx_d)  "dotwx_ref"
  Sum/1 -> wy_control/1
  wy_control/1 -> MATLAB Function/3(My_d)  "dotwy_ref"
  wz_control/1 -> MATLAB Function/4(Mz_d)  "dotwz_ref"
  Sum2/1 -> wz_control/1
  attitude_d/1 -> MATLAB Function1/2(euler_d)
  Bus Selector3/2 -> attrates_ref_selector/2(arm)  "<arm>"
  Bus Selector3/1 -> attrates_ref_selector/1(flight_mode)  "<flight_mode>"
  Bus Selector3/3 -> attrates_ref_selector/3(ctrl_mode)  "<ctrl_mode>"
  vehicle_mode/1 -> Bus Selector3/1
  attrates_ref_selector/1(rate_ctrl_integral_reset) -> Selector1/1, Selector2/1, Selector3/1

== system LW_ctrl/Controller/PID_Controller/PID_Controller/local_pos_ref_selector ==
  StatesRef : Inport
  vehicle_mode : Inport  Port=2
  VehicleStates : Inport  Port=3
  Bus Creator : BusCreator  Inputs=5
  Bus Selector1 : BusSelector  OutputSignals=vehicle_local_position.timestamp,vehicle_local_position.vehicle_local_pos,vehicle_local_position.vehicle_local_vel,vehicle_local_position.delta_xy,vehicle_local_position.xy_reset_counter,vehicle_local_position.delta_z,vehicle_local_position.z_reset_counter,vehicle_local_position.delta_vxy,vehicle_local_position.vxy_reset_counter,vehicle_local_position.delta_vz,vehicle_local_position.vz_reset_counter,vehicle_local_position.delta_heading,vehicle_local_position.heading_reset_counter,vehicle_attitude.quat,vehicle_attitude.omega,states_flag,vehicle_attitude.dm_est
  Bus Selector2 : BusSelector  OutputSignals=ctrl_mode,flight_mode,arm
  Bus Selector3 : BusSelector  OutputSignals=manual.vel_ref,manual.rates_ref,offboard
  nan_inf_mode : MATLAB Function  TreatAsAtomicUnit=on
  nan_inf_mode1 : MATLAB Function  TreatAsAtomicUnit=on
  position control : MATLAB Function  TreatAsAtomicUnit=on
  local_pos_ref : Outport
  wires:
  vehicle_mode/1 -> Bus Selector2/1
  VehicleStates/1 -> Bus Selector1/1
  Bus Selector1/2 -> position control/5(vehicle_pos)  "<vehicle_local_pos>"
  Bus Selector1/3 -> position control/6(vehicle_vel)  "<vehicle_local_vel>"
  StatesRef/1 -> Bus Selector3/1
  Bus Selector3/3 -> position control/3(offboard_ref)  "<offboard>"
  Bus Selector3/1 -> position control/1(manual_vel_ref)  "<vel_ref>"
  nan_inf_mode/1(y) -> position control/21(ctrl_mode)
  nan_inf_mode1/1(y) -> position control/22(flight_mode)
  Bus Selector2/1 -> nan_inf_mode/1(u)  "<ctrl_mode>"
  Bus Selector2/2 -> nan_inf_mode1/1(u)  "<flight_mode>"
  Bus Selector1/14 -> position control/17(q)  "<quat>"
  Bus Selector3/2 -> position control/2(manual_rates_ref)  "<rates_ref>"
  position control/3(yaw_ref) -> Bus Creator/3
  position control/1(pos_ref) -> Bus Creator/1
  position control/2(vd_lim) -> Bus Creator/2
  Bus Creator/1 -> local_pos_ref/1
  Bus Selector1/1 -> position control/4(timestamp)  "<timestamp>"
  Bus Selector1/16 -> position control/19(states_flag)  "<states_flag>"
  position control/5(man_acc_ff) -> Bus Creator/5
  Bus Selector2/3 -> position control/23(arm)  "<arm>"
  Bus Selector1/4 -> position control/7(delta_xy)  "<delta_xy>"
  Bus Selector1/5 -> position control/8(xy_reset_counter)  "<xy_reset_counter>"
  Bus Selector1/6 -> position control/9(delta_z)  "<delta_z>"
  Bus Selector1/7 -> position control/10(z_reset_counter)  "<z_reset_counter>"
  Bus Selector1/8 -> position control/11(delta_vxy)  "<delta_vxy>"
  Bus Selector1/9 -> position control/12(vxy_reset_counter)  "<vxy_reset_counter>"
  Bus Selector1/10 -> position control/13(delta_vz)  "<delta_vz>"
  Bus Selector1/11 -> position control/14(vz_reset_counter)  "<vz_reset_counter>"
  Bus Selector1/12 -> position control/15(delta_heading)  "<delta_heading>"
  Bus Selector1/13 -> position control/16(heading_reset_counter)  "<heading_reset_counter>"
  Bus Selector1/17 -> position control/20(dm_est)  "<dm_est>"
  Bus Selector1/15 -> position control/18(wb)  "<omega>"
  position control/4(wbz_ref) -> Bus Creator/4

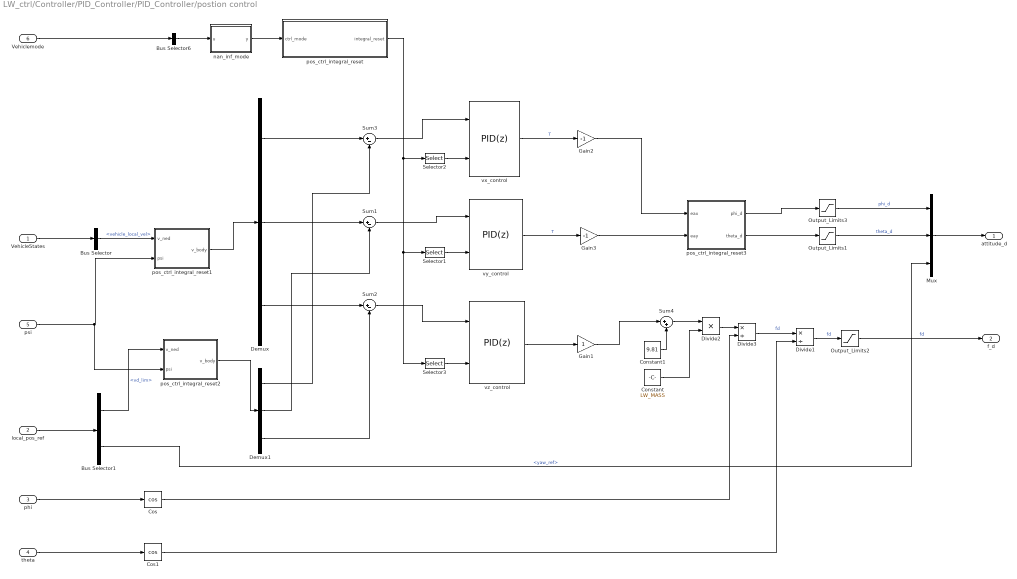
== system LW_ctrl/Controller/PID_Controller/PID_Controller/postion control ==
  VehicleStates : Inport
  local_pos_ref : Inport  Port=2
  phi : Inport  Port=3
  theta : Inport  Port=4
  psi : Inport  Port=5
  Vehiclemode : Inport  Port=6
  Bus Selector : BusSelector  OutputSignals=vehicle_local_position.vehicle_local_vel
  Bus Selector1 : BusSelector  OutputSignals=vd_lim,yaw_ref
  Bus Selector6 : BusSelector  OutputSignals=ctrl_mode,arm  OutputAsBus=on
  Constant : Constant  Value=LW_MASS
  Constant1 : Constant  Value=9.81
  Cos : Trigonometry  Operator=cos
  Cos1 : Trigonometry  Operator=cos
  Demux : Demux  Outputs=3
  Demux1 : Demux  Outputs=3
  Divide1 : Product  Inputs=*/
  Divide2 : Product  Inputs=**
  Divide3 : Product  Inputs=*/
  Gain1 : Gain
  Gain2 : Gain  Gain=-1
  Gain3 : Gain  Gain=-1
  Mux : Mux  Inputs=3
  Output_Limits1 : Saturate  UpperLimit=20/180*pi  LowerLimit=-20/180*pi
  Output_Limits2 : Saturate  UpperLimit=40  LowerLimit=0
  Output_Limits3 : Saturate  UpperLimit=20/180*pi  LowerLimit=-20/180*pi
  Selector1 : Selector  InputPortWidth=2  IndexOptions=Index vector (dialog)  Indices=[1]  OutputSizes=1
  Selector2 : Selector  InputPortWidth=2  IndexOptions=Index vector (dialog)  Indices=[1]  OutputSizes=1
  Selector3 : Selector  InputPortWidth=2  IndexOptions=Index vector (dialog)  Indices=[2]  OutputSizes=1
  Sum1 : Sum  Inputs=|+-
  Sum2 : Sum  Inputs=|+-
  Sum3 : Sum  Inputs=|+-
  Sum4 : Sum  Inputs=|++
  nan_inf_mode : MATLAB Function  TreatAsAtomicUnit=on
  pos_ctrl_integral_reset : MATLAB Function  TreatAsAtomicUnit=on
  pos_ctrl_integral_reset1 : MATLAB Function  TreatAsAtomicUnit=on
  pos_ctrl_integral_reset2 : MATLAB Function  TreatAsAtomicUnit=on
  pos_ctrl_integral_reset3 : MATLAB Function  TreatAsAtomicUnit=on
  vx_control : slpidlib/PID Controller  Controller=PID  Form=Parallel  TimeDomain=Discrete-time  UseExternalTs=off  SampleTime=-1  IntegratorMethod=Forward Euler  FilterMethod=Forward Euler  ControllerParametersSource=internal  P=3  I=0  UseKiTs=off  D=0  UseExternalDerivativeSource=off  N=100  UseFilter=on  TunerSelectOption=Transfer Function Based (PID Tuner App)  InitialConditionSource=internal  InitialConditionForIntegrator=0  InitialConditionForFilter=0  DifferentiatorICPrevScaledInput=0  ExternalReset=level  TrackingMode=off  Kt=1  LimitOutput=on  SatLimitsSource=internal  UpperSaturationLimit=LW_X_ACCEL_MAX  LowerSaturationLimit=LW_X_ACCEL_MIN  LinearizeAsGain=off  AntiWindupMode=clamping  Kb=1  LimitIntegrator=off  UpperIntegratorSaturationLimit=inf  LowerIntegratorSaturationLimit=-inf  POutMin=[]  POutMax=[]  IOutMin=[]  IOutMax=[]  DOutMin=[]  DOutMax=[]  NOutMin=[]  NOutMax=[]  SumOutMin=[]  SumOutMax=[]  SaturationOutMin=[]  SaturationOutMax=[]  PParamMin=[]  PParamMax=[]  IParamMin=[]  IParamMax=[]  DParamMin=[]  DParamMax=[]  NParamMin=[]  NParamMax=[]  KbParamMin=[]  KbParamMax=[]  KtParamMin=[]  KtParamMax=[]  KbOutMin=[]  KbOutMax=[]  KtOutMin=[]  KtOutMax=[]  IntegratorOutMin=-2.2  IntegratorOutMax=2.2  FilterOutMin=[]  FilterOutMax=[]  SumI1OutMin=[]  SumI1OutMax=[]  SumI2OutMin=[]  SumI2OutMax=[]  SumI3OutMin=[]  SumI3OutMax=[]  SumI4OutMin=[]  SumI4OutMax=[]  SumDOutMin=[]  SumDOutMax=[]  DifferentiatorOutMin=[]  DifferentiatorOutMax=[]  FilterDiffOutCoefMin=[]  FilterDiffOutCoefMax=[]  ReciprocalOutMin=[]  ReciprocalOutMax=[]  SumDenOutMin=[]  SumDenOutMax=[]  SumNumOutMin=[]  SumNumOutMax=[]  DivideOutMin=[]  DivideOutMax=[]  UdiffTsProdOutMin=[]  UdiffTsProdOutMax=[]  NTsProdOutMin=[]  NTsProdOutMax=[]  UintegralTsProdOutMin=[]  UintegralTsProdOutMax=[]  UngainTsProdOutMin=[]  UngainTsProdOutMax=[]  ClampingZeroOutDataTypeStr=Inherit: Inherit via back propagation  ClampingZeroOutMin=[]  ClampingZeroOutMax=[]  FilterDenConstantOutDataTypeStr=Inherit: Inherit via back propagation  FilterDenConstantOutMin=[]  FilterDenConstantOutMax=[]  PCopyOutDataTypeStr=Inherit: Inherit via back propagation  PCopyOutMin=[]  PCopyOutMax=[]  NCopyOutDataTypeStr=Inherit: Inherit via back propagation  NCopyOutMin=[]  NCopyOutMax=[]  IntegratorContinuousStateAttributes=''  IntegratorStateMustResolveToSignalObject=off  IntegratorRTWStateStorageClass=Auto  FilterContinuousStateAttributes=''  FilterStateMustResolveToSignalObject=off  FilterRTWStateStorageClass=Auto  ParallelPVariant=InternalParameters  IdealPVariant=Disabled  IVariant=InternalParameters  DVariant=InternalParameters  IntegratorVariant=Discrete  SatVariant=Enabled  AWVariant=DiscClampingParallel  PCopyVariant=Disabled  TRVariant=Disabled  FdbkBlocksVariant=Forward  IdealPFdbkVariant=Disabled  SatFdbkVariant=Disabled  DerivativeFilterVariant=ForwardEulerFilter  NVariant=InternalParameters  NCopyVariant=Disabled  FilterICVariant=InternalICsFilter  IntegratorICVariant=InternalICs  ExternalResetVariant=ExternalReset  TRSumVariant=Passthrough  SumFdbkVariant=Disabled  SumVariant=Sum_PID  TsampFilterVariant=InternalTs  TsampNgainVariant=Passthrough  TsampIntegralVariant=Disabled_SignalSpec  ExternalSaturationOutDataTypeStr=Inherit: Same as second input  DerivativeSourceVariant=ErrorSignal  PreIntVariant=InternalPreInt
  vy_control : slpidlib/PID Controller  Controller=PID  Form=Parallel  TimeDomain=Discrete-time  UseExternalTs=off  SampleTime=-1  IntegratorMethod=Forward Euler  FilterMethod=Forward Euler  ControllerParametersSource=internal  P=3  I=0  UseKiTs=off  D=0  UseExternalDerivativeSource=off  N=100  UseFilter=on  TunerSelectOption=Transfer Function Based (PID Tuner App)  InitialConditionSource=internal  InitialConditionForIntegrator=0  InitialConditionForFilter=0  DifferentiatorICPrevScaledInput=0  ExternalReset=level  TrackingMode=off  Kt=1  LimitOutput=on  SatLimitsSource=internal  UpperSaturationLimit=LW_Y_ACCEL_MAX  LowerSaturationLimit=LW_Y_ACCEL_MIN  LinearizeAsGain=off  AntiWindupMode=clamping  Kb=1  LimitIntegrator=off  UpperIntegratorSaturationLimit=inf  LowerIntegratorSaturationLimit=-inf  POutMin=[]  POutMax=[]  IOutMin=[]  IOutMax=[]  DOutMin=[]  DOutMax=[]  NOutMin=[]  NOutMax=[]  SumOutMin=[]  SumOutMax=[]  SaturationOutMin=[]  SaturationOutMax=[]  PParamMin=[]  PParamMax=[]  IParamMin=[]  IParamMax=[]  DParamMin=[]  DParamMax=[]  NParamMin=[]  NParamMax=[]  KbParamMin=[]  KbParamMax=[]  KtParamMin=[]  KtParamMax=[]  KbOutMin=[]  KbOutMax=[]  KtOutMin=[]  KtOutMax=[]  IntegratorOutMin=-2.2  IntegratorOutMax=2.2  FilterOutMin=[]  FilterOutMax=[]  SumI1OutMin=[]  SumI1OutMax=[]  SumI2OutMin=[]  SumI2OutMax=[]  SumI3OutMin=[]  SumI3OutMax=[]  SumI4OutMin=[]  SumI4OutMax=[]  SumDOutMin=[]  SumDOutMax=[]  DifferentiatorOutMin=[]  DifferentiatorOutMax=[]  FilterDiffOutCoefMin=[]  FilterDiffOutCoefMax=[]  ReciprocalOutMin=[]  ReciprocalOutMax=[]  SumDenOutMin=[]  SumDenOutMax=[]  SumNumOutMin=[]  SumNumOutMax=[]  DivideOutMin=[]  DivideOutMax=[]  UdiffTsProdOutMin=[]  UdiffTsProdOutMax=[]  NTsProdOutMin=[]  NTsProdOutMax=[]  UintegralTsProdOutMin=[]  UintegralTsProdOutMax=[]  UngainTsProdOutMin=[]  UngainTsProdOutMax=[]  ClampingZeroOutDataTypeStr=Inherit: Inherit via back propagation  ClampingZeroOutMin=[]  ClampingZeroOutMax=[]  FilterDenConstantOutDataTypeStr=Inherit: Inherit via back propagation  FilterDenConstantOutMin=[]  FilterDenConstantOutMax=[]  PCopyOutDataTypeStr=Inherit: Inherit via back propagation  PCopyOutMin=[]  PCopyOutMax=[]  NCopyOutDataTypeStr=Inherit: Inherit via back propagation  NCopyOutMin=[]  NCopyOutMax=[]  IntegratorContinuousStateAttributes=''  IntegratorStateMustResolveToSignalObject=off  IntegratorRTWStateStorageClass=Auto  FilterContinuousStateAttributes=''  FilterStateMustResolveToSignalObject=off  FilterRTWStateStorageClass=Auto  ParallelPVariant=InternalParameters  IdealPVariant=Disabled  IVariant=InternalParameters  DVariant=InternalParameters  IntegratorVariant=Discrete  SatVariant=Enabled  AWVariant=DiscClampingParallel  PCopyVariant=Disabled  TRVariant=Disabled  FdbkBlocksVariant=Forward  IdealPFdbkVariant=Disabled  SatFdbkVariant=Disabled  DerivativeFilterVariant=ForwardEulerFilter  NVariant=InternalParameters  NCopyVariant=Disabled  FilterICVariant=InternalICsFilter  IntegratorICVariant=InternalICs  ExternalResetVariant=ExternalReset  TRSumVariant=Passthrough  SumFdbkVariant=Disabled  SumVariant=Sum_PID  TsampFilterVariant=InternalTs  TsampNgainVariant=Passthrough  TsampIntegralVariant=Disabled_SignalSpec  ExternalSaturationOutDataTypeStr=Inherit: Same as second input  DerivativeSourceVariant=ErrorSignal  PreIntVariant=InternalPreInt
  vz_control : slpidlib/PID Controller  Controller=PID  Form=Parallel  TimeDomain=Discrete-time  UseExternalTs=off  SampleTime=-1  IntegratorMethod=Forward Euler  FilterMethod=Forward Euler  ControllerParametersSource=internal  P=5.5  I=0.3  UseKiTs=off  D=0  UseExternalDerivativeSource=off  N=100  UseFilter=on  TunerSelectOption=Transfer Function Based (PID Tuner App)  InitialConditionSource=internal  InitialConditionForIntegrator=0  InitialConditionForFilter=0  DifferentiatorICPrevScaledInput=0  ExternalReset=level  TrackingMode=off  Kt=1  LimitOutput=on  SatLimitsSource=internal  UpperSaturationLimit=LW_Z_ACCEL_UP  LowerSaturationLimit=LW_Z_ACCEL_LOW  LinearizeAsGain=off  AntiWindupMode=clamping  Kb=1  LimitIntegrator=off  UpperIntegratorSaturationLimit=inf  LowerIntegratorSaturationLimit=-inf  POutMin=[]  POutMax=[]  IOutMin=[]  IOutMax=[]  DOutMin=[]  DOutMax=[]  NOutMin=[]  NOutMax=[]  SumOutMin=[]  SumOutMax=[]  SaturationOutMin=[]  SaturationOutMax=[]  PParamMin=[]  PParamMax=[]  IParamMin=[]  IParamMax=[]  DParamMin=[]  DParamMax=[]  NParamMin=[]  NParamMax=[]  KbParamMin=[]  KbParamMax=[]  KtParamMin=[]  KtParamMax=[]  KbOutMin=[]  KbOutMax=[]  KtOutMin=[]  KtOutMax=[]  IntegratorOutMin=Saturation_I_AZ_LOW  IntegratorOutMax=Saturation_I_AZ_UP  FilterOutMin=[]  FilterOutMax=[]  SumI1OutMin=[]  SumI1OutMax=[]  SumI2OutMin=[]  SumI2OutMax=[]  SumI3OutMin=[]  SumI3OutMax=[]  SumI4OutMin=[]  SumI4OutMax=[]  SumDOutMin=[]  SumDOutMax=[]  DifferentiatorOutMin=[]  DifferentiatorOutMax=[]  FilterDiffOutCoefMin=[]  FilterDiffOutCoefMax=[]  ReciprocalOutMin=[]  ReciprocalOutMax=[]  SumDenOutMin=[]  SumDenOutMax=[]  SumNumOutMin=[]  SumNumOutMax=[]  DivideOutMin=[]  DivideOutMax=[]  UdiffTsProdOutMin=[]  UdiffTsProdOutMax=[]  NTsProdOutMin=[]  NTsProdOutMax=[]  UintegralTsProdOutMin=[]  UintegralTsProdOutMax=[]  UngainTsProdOutMin=[]  UngainTsProdOutMax=[]  ClampingZeroOutDataTypeStr=Inherit: Inherit via back propagation  ClampingZeroOutMin=[]  ClampingZeroOutMax=[]  FilterDenConstantOutDataTypeStr=Inherit: Inherit via back propagation  FilterDenConstantOutMin=[]  FilterDenConstantOutMax=[]  PCopyOutDataTypeStr=Inherit: Inherit via back propagation  PCopyOutMin=[]  PCopyOutMax=[]  NCopyOutDataTypeStr=Inherit: Inherit via back propagation  NCopyOutMin=[]  NCopyOutMax=[]  IntegratorContinuousStateAttributes=''  IntegratorStateMustResolveToSignalObject=off  IntegratorRTWStateStorageClass=Auto  FilterContinuousStateAttributes=''  FilterStateMustResolveToSignalObject=off  FilterRTWStateStorageClass=Auto  ParallelPVariant=InternalParameters  IdealPVariant=Disabled  IVariant=InternalParameters  DVariant=InternalParameters  IntegratorVariant=Discrete  SatVariant=Enabled  AWVariant=DiscClampingParallel  PCopyVariant=Disabled  TRVariant=Disabled  FdbkBlocksVariant=Forward  IdealPFdbkVariant=Disabled  SatFdbkVariant=Disabled  DerivativeFilterVariant=ForwardEulerFilter  NVariant=InternalParameters  NCopyVariant=Disabled  FilterICVariant=InternalICsFilter  IntegratorICVariant=InternalICs  ExternalResetVariant=ExternalReset  TRSumVariant=Passthrough  SumFdbkVariant=Disabled  SumVariant=Sum_PID  TsampFilterVariant=InternalTs  TsampNgainVariant=Passthrough  TsampIntegralVariant=Disabled_SignalSpec  ExternalSaturationOutDataTypeStr=Inherit: Same as second input  DerivativeSourceVariant=ErrorSignal  PreIntVariant=InternalPreInt
  attitude_d : Outport
  f_d : Outport  Port=2
  wires:
  Constant/1 -> Divide2/2
  Sum3/1 -> vx_control/1
  Sum1/1 -> vy_control/1
  Sum2/1 -> vz_control/1
  Constant1/1 -> Sum4/2
  vz_control/1 -> Gain1/1
  vy_control/1 -> Gain3/1  "T"
  vx_control/1 -> Gain2/1  "T"
  Sum4/1 -> Divide2/1
  Gain1/1 -> Sum4/1
  Divide2/1 -> Divide3/1
  Divide3/1 -> Divide1/1  "fd"
  Divide1/1 -> Output_Limits2/1  "fd"
  pos_ctrl_integral_reset3/1(phi_d) -> Output_Limits3/1
  pos_ctrl_integral_reset3/2(theta_d) -> Output_Limits1/1
  Demux/1 -> Sum3/1
  Demux/3 -> Sum2/1
  Demux/2 -> Sum1/1
  local_pos_ref/1 -> Bus Selector1/1
  Demux1/3 -> Sum2/2
  phi/1 -> Cos/1
  theta/1 -> Cos1/1
  Cos/1 -> Divide3/2
  Cos1/1 -> Divide1/2
  Bus Selector1/2 -> Mux/3  "<yaw_ref>"
  VehicleStates/1 -> Bus Selector/1
  Bus Selector1/1 -> pos_ctrl_integral_reset2/1(v_ned)  "<vd_lim>"
  pos_ctrl_integral_reset2/1(v_body) -> Demux1/1
  Bus Selector/1 -> pos_ctrl_integral_reset1/1(v_ned)  "<vehicle_local_vel>"
  psi/1 -> pos_ctrl_integral_reset2/2(psi), pos_ctrl_integral_reset1/2(psi)
  Gain2/1 -> pos_ctrl_integral_reset3/1(eax)
  Gain3/1 -> pos_ctrl_integral_reset3/2(eay)
  Demux1/1 -> Sum3/2
  Demux1/2 -> Sum1/2
  Output_Limits3/1 -> Mux/1  "phi_d"
  Output_Limits1/1 -> Mux/2  "theta_d"
  Mux/1 -> attitude_d/1
  Vehiclemode/1 -> Bus Selector6/1
  Bus Selector6/1 -> nan_inf_mode/1(u)
  nan_inf_mode/1(y) -> pos_ctrl_integral_reset/1(ctrl_mode)
  Selector2/1 -> vx_control/2
  Selector1/1 -> vy_control/2
  Selector3/1 -> vz_control/2
  pos_ctrl_integral_reset/1(integral_reset) -> Selector2/1, Selector3/1, Selector1/1
  Output_Limits2/1 -> f_d/1  "fd"
  pos_ctrl_integral_reset1/1(v_body) -> Demux/1

== system LW_ctrl/Controller/PID_Controller/PID_Controller/select parameter ==
  VehicleStates : Inport
  Bus Selector : BusSelector  OutputSignals=vehicle_attitude.quat,vehicle_attitude.omega
  Demux2 : Demux  Outputs=3
  Demux3 : Demux  Outputs=3
  MATLAB Function : MATLAB Function  TreatAsAtomicUnit=on
  theta : Outport
  phi : Outport  Port=2
  wx : Outport  Port=3
  wy : Outport  Port=4
  wz : Outport  Port=5
  psi : Outport  Port=6
  quat : Outport  Port=7
  wires:
  Demux3/1 -> phi/1
  Demux2/2 -> wy/1  "wy"
  Demux2/1 -> wx/1
  Demux2/3 -> wz/1
  Demux3/2 -> theta/1
  Demux3/3 -> psi/1
  VehicleStates/1 -> Bus Selector/1
  Bus Selector/1 -> quat/1, MATLAB Function/1(u)  "<quat>"
  Bus Selector/2 -> Demux2/1  "<omega>"
  MATLAB Function/1(y) -> Demux3/1
